simulink model "jointSpaceTrajController_InitContext1"  (Simulink 8.0)
settings: Solver=FixedStepDiscrete  StartTime=0.0  StopTime=2.0  FixedStep=Ts  RelTol=1e-3
libraries: WBCLibrary x4
settings Model: Creator=nunoguedelha  LastModifiedBy=nunoguedelha

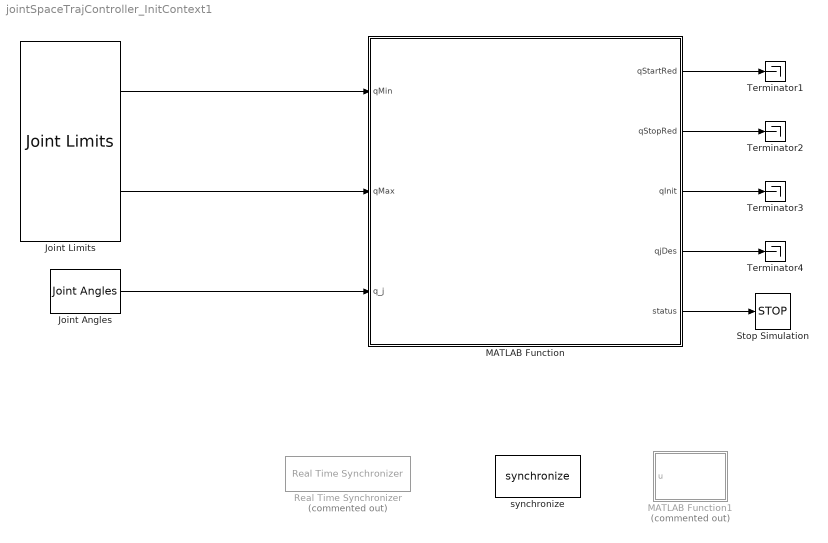
== system jointSpaceTrajController_InitContext1 ==
  Joint Angles : WBCLibrary/wholeBodyStates/Joint Angles  robotName=robotName  localName=localName
  Joint Limits : WBCLibrary/wholeBodyModel/Joint Limits  robotName=robotName  localName=localName
  MATLAB Function : MATLAB Function  TreatAsAtomicUnit=on
  MATLAB Function1 : MATLAB Function  Commented=on  TreatAsAtomicUnit=on
  Real Time Synchronizer : WBCLibrary/Utilities/Real Time Synchronizer  Priority=-10  Commented=on  threadPeriod=Ts
  Stop Simulation : Stop
  Terminator{1..4} (4 alike) : Terminator
  synchronize : WBCLibrary/Utilities/synchronize  rate=0.010  scaleFactor=1
  wires:
  Joint Limits/1 -> MATLAB Function/1(qMin)
  Joint Limits/2 -> MATLAB Function/2(qMax)
  Joint Angles/1 -> MATLAB Function/3(q_j)
  MATLAB Function/1(qStartRed) -> Terminator1/1
  MATLAB Function/2(qStopRed) -> Terminator2/1
  MATLAB Function/3(qInit) -> Terminator3/1
  MATLAB Function/5(status) -> Stop Simulation/1
  MATLAB Function/4(qjDes) -> Terminator4/1

== matlab function MATLAB Function ==
  data: qMin input double; qMax input double; qStartRed output double; qStopRed output double; q_j input double; qInit output double; qjDes output double; status output double
function [qStartRed, qStopRed, qInit, qjDes, status] = initTrajParams(qMin, qMax, q_j)
%#codegen

% just return q_j for saving it to the workspace
qInit = q_j;
qjDes = q_j;

%% adjusted joint limits.
%
% First, choose the limits in order to avoid collisions: we can just assign
% opposite limits between legs, then arms, etc.
% torso = [1:3];
% leftArm = [4:7];
% rightArm = [8:11];
% leftLeg = [12:17];
% rightLeg = [18:23];
% qStart = [qMin(torso) ; qMin(leftArm) ; qMax(rightArm) ; qMin(leftLeg) ; qMax(rightLeg)];
% qStop  = [qMax(torso) ; qMax(leftArm) ; qMin(rightArm) ; qMax(leftLeg) ; qMin(rightLeg)];

leftArm = 1:4;
rightArm = 5:8;
leftLeg = 9:14;
rightLeg = 15:20;

% For the min boundary (qMin), we shift by 2deg in the direction qMin->qMax.
% For the max boundary (qMax), we shift by 2deg in the direction qMax->qMin.
DeltaQ = qMax - qMin;
qMinRed = qMin + DeltaQ*0.15; % 1/10th of the trajectory span
qMaxRed = qMax - DeltaQ*0.3;
% specific to iCubGenova02
qMinRed(leftLeg(2)) = qMin(leftLeg(2)) + (32*pi/180); % +32 degrees
qMinRed(rightLeg(2)) = qMin(rightLeg(2)) + (32*pi/180); % +32 degrees

% Reorder boundaries for generating disymetric trajectories
qStartRed = [qMinRed(leftArm) ; qMinRed(rightArm) ; qMinRed(leftLeg) ; qMinRed(rightLeg)];
qStopRed  = [qMaxRed(leftArm) ; qMaxRed(rightArm) ; qMaxRed(leftLeg) ; qMaxRed(rightLeg)];


% set status to 1 to stop simulation
status = 1;

== matlab function MATLAB Function1 ==
  data: u input double
function mySimOut(u)
%#codegen
coder.extrinsic('assignin');
assignin('base','q_j', u);
